simulink model "banc_test_bras_brushless_PF35_couronne_grande"  (R2025a)
settings: Solver=daessc  StartTime=0.0  StopTime=40  FixedStep=Ts  RelTol=1e-3  EnableMultiTasking=on
undefined symbols (not defined in the file or in its folder): Connection1, Connection10, Connection11, Connection12, Connection2, Connection3, Connection4, Connection5, Connection6, Connection7, Connection8, Connection9, X, Y, Z
libraries: sm_lib x16, nesl_utility x4
settings Model: Creator=vincp  LastModifiedBy=VincentPERRET
settings SolverCC: MaxConsecutiveMinStep=100  AllowMultiTaskInputOutput=on  ZeroCrossAlgorithm=Adaptive  PositivePriorityOrder=on
settings DataIOCC: ReturnWorkspaceOutputsName=tp821c331c_e25c_45d9_bd23_b4f1d96f521a
settings DebuggingCC: IgnoredZcDiagnostic=none
settings SFSimCC: SimTargetLang=C++  SimDLTargetLibrary=mkl-dnn
settings RTWCC: GPUComputeCapability=3.5
settings SimscapeCC: ExplicitSolverDiagnosticOptions=none  SimscapeLogName=simlog_ee_bldc_speed_control  SimscapeLogLimitData=off

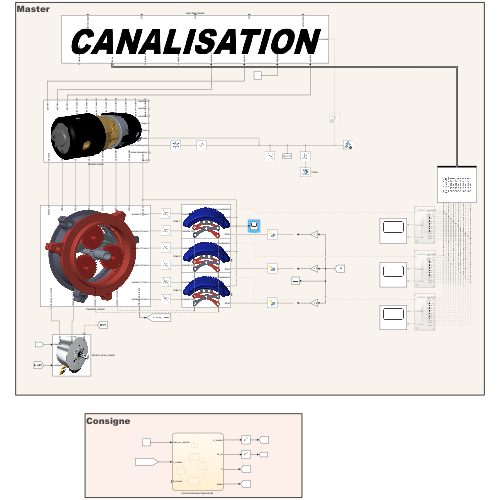
[thumbnail: Simulink's stored preview of the top-level diagram]
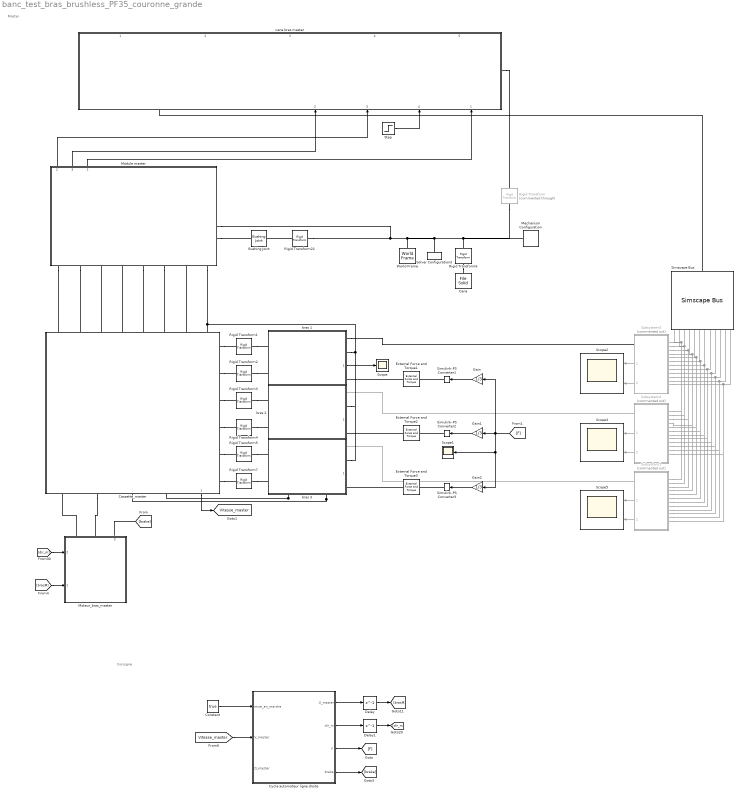
== system banc_test_bras_brushless_PF35_couronne_grande ==
  note: Consigne
  note: Master
  Bushing Joint : sm_lib/Joints/Bushing Joint  JointMode=Normal  CompositeWrenchDir=FollowerOnBase  CompositeWrenchFrame=BaseFrame  SenseConstraintForce=off  SenseConstraintTorque=off  SenseTotalForce=off  SenseTotalTorque=off  PxPositionTargetSpecify=off  PxPositionTargetPriority=High  PxPositionTargetValue=0  PxPositionTargetValueUnits=m  PxVelocityTargetSpecify=off  PxVelocityTargetPriority=High  PxVelocityTargetValue=0  PxVelocityTargetValueUnits=m/s  PxEquilibriumPosition=0  PxEquilibriumPositionUnits=m  PxSpringStiffness=0  PxSpringStiffnessUnits=N/m  PxDampingCoefficient=0  PxDampingCoefficientUnits=N/(m/s)  PxLowerLimitSpecify=off  PxLowerLimitBound=-1  PxLowerLimitBoundUnits=m  PxLowerLimitStiffness=1e6  PxLowerLimitStiffnessUnits=N/m  PxLowerLimitDamping=1e3  PxLowerLimitDampingUnits=N/(m/s)  PxLowerLimitTransitionRegionWidth=1e-4  PxLowerLimitTransitionRegionWidthUnits=m  PxUpperLimitSpecify=off  PxUpperLimitBound=1  PxUpperLimitBoundUnits=m  PxUpperLimitStiffness=1e6  PxUpperLimitStiffnessUnits=N/m  PxUpperLimitDamping=1e3  PxUpperLimitDampingUnits=N/(m/s)  PxUpperLimitTransitionRegionWidth=1e-4  PxUpperLimitTransitionRegionWidthUnits=m  PxTorqueActuationMode=NoTorque  PxMotionActuationMode=ComputedMotion  PxSensePosition=off  PxSenseVelocity=off  PxSenseAcceleration=off  PxSenseTorqueForce=off  PxSenseLowerLimitTorqueForce=off  PxSenseUpperLimitTorqueForce=off  PyPositionTargetSpecify=off  PyPositionTargetPriority=High  PyPositionTargetValue=0  PyPositionTargetValueUnits=m  PyVelocityTargetSpecify=off  PyVelocityTargetPriority=High  PyVelocityTargetValue=0  PyVelocityTargetValueUnits=m/s  PyEquilibriumPosition=0  PyEquilibriumPositionUnits=m  PySpringStiffness=0  PySpringStiffnessUnits=N/m  PyDampingCoefficient=0  PyDampingCoefficientUnits=N/(m/s)  PyLowerLimitSpecify=off  PyLowerLimitBound=-1  PyLowerLimitBoundUnits=m  PyLowerLimitStiffness=1e6  PyLowerLimitStiffnessUnits=N/m  PyLowerLimitDamping=1e3  PyLowerLimitDampingUnits=N/(m/s)  PyLowerLimitTransitionRegionWidth=1e-4  PyLowerLimitTransitionRegionWidthUnits=m  PyUpperLimitSpecify=off  PyUpperLimitBound=1  PyUpperLimitBoundUnits=m  PyUpperLimitStiffness=1e6  PyUpperLimitStiffnessUnits=N/m  PyUpperLimitDamping=1e3  PyUpperLimitDampingUnits=N/(m/s)  PyUpperLimitTransitionRegionWidth=1e-4  PyUpperLimitTransitionRegionWidthUnits=m  PyTorqueActuationMode=NoTorque  PyMotionActuationMode=ComputedMotion  PySensePosition=off  PySenseVelocity=off  PySenseAcceleration=off  PySenseTorqueForce=off  PySenseLowerLimitTorqueForce=off  PySenseUpperLimitTorqueForce=off  PzPositionTargetSpecify=off  PzPositionTargetPriority=High  PzPositionTargetValue=0  PzPositionTargetValueUnits=m  PzVelocityTargetSpecify=off  PzVelocityTargetPriority=High  PzVelocityTargetValue=-0.1  PzVelocityTargetValueUnits=m/s  PzEquilibriumPosition=0  PzEquilibriumPositionUnits=m  PzSpringStiffness=0  PzSpringStiffnessUnits=N/m  PzDampingCoefficient=0  PzDampingCoefficientUnits=N/(m/s)  PzLowerLimitSpecify=off  PzLowerLimitBound=-1  PzLowerLimitBoundUnits=m  PzLowerLimitStiffness=1e6  PzLowerLimitStiffnessUnits=N/m  PzLowerLimitDamping=1e3  PzLowerLimitDampingUnits=N/(m/s)  PzLowerLimitTransitionRegionWidth=1e-4  PzLowerLimitTransitionRegionWidthUnits=m  PzUpperLimitSpecify=off  PzUpperLimitBound=1  PzUpperLimitBoundUnits=m  PzUpperLimitStiffness=1e6  PzUpperLimitStiffnessUnits=N/m  PzUpperLimitDamping=1e3  PzUpperLimitDampingUnits=N/(m/s)  PzUpperLimitTransitionRegionWidth=1e-4  PzUpperLimitTransitionRegionWidthUnits=m  PzTorqueActuationMode=NoTorque  PzMotionActuationMode=ComputedMotion  PzSensePosition=off  PzSenseVelocity=off  PzSenseAcceleration=off  PzSenseTorqueForce=off  PzSenseLowerLimitTorqueForce=off  PzSenseUpperLimitTorqueForce=off  RxPositionTargetSpecify=off  RxPositionTargetPriority=High  RxPositionTargetValue=0  RxPositionTargetValueUnits=deg  RxVelocityTargetSpecify=off  RxVelocityTargetPriority=High  RxVelocityTargetValue=0  RxVelocityTargetValueUnits=deg/s  RxEquilibriumPosition=0  RxEquilibriumPositionUnits=deg  RxSpringStiffness=0  RxSpringStiffnessUnits=N*m/deg  RxDampingCoefficient=0  RxDampingCoefficientUnits=N*m/(deg/s)  RxLowerLimitSpecify=off  RxLowerLimitBound=-90  RxLowerLimitBoundUnits=deg  RxLowerLimitStiffness=1e4  RxLowerLimitStiffnessUnits=N*m/deg  RxLowerLimitDamping=10  RxLowerLimitDampingUnits=N*m/(deg/s)  RxLowerLimitTransitionRegionWidth=0.1  RxLowerLimitTransitionRegionWidthUnits=deg  RxUpperLimitSpecify=off  RxUpperLimitBound=90  RxUpperLimitBoundUnits=deg  RxUpperLimitStiffness=1e4  RxUpperLimitStiffnessUnits=N*m/deg  RxUpperLimitDamping=10  RxUpperLimitDampingUnits=N*m/(deg/s)  RxUpperLimitTransitionRegionWidth=0.1  RxUpperLimitTransitionRegionWidthUnits=deg  RxTorqueActuationMode=NoTorque  RxMotionActuationMode=ComputedMotion  RxSensePosition=off  RxSenseVelocity=off  RxSenseAcceleration=off  RxSenseTorqueForce=off  RxSenseLowerLimitTorqueForce=off  RxSenseUpperLimitTorqueForce=off  RyPositionTargetSpecify=off  RyPositionTargetPriority=High  RyPositionTargetValue=0  RyPositionTargetValueUnits=deg  RyVelocityTargetSpecify=off  RyVelocityTargetPriority=High  RyVelocityTargetValue=0  RyVelocityTargetValueUnits=deg/s  RyEquilibriumPosition=0  RyEquilibriumPositionUnits=deg  RySpringStiffness=0  RySpringStiffnessUnits=N*m/deg  RyDampingCoefficient=0  RyDampingCoefficientUnits=N*m/(deg/s)  RyLowerLimitSpecify=off  RyLowerLimitBound=-90  RyLowerLimitBoundUnits=deg  RyLowerLimitStiffness=1e4  RyLowerLimitStiffnessUnits=N*m/deg  RyLowerLimitDamping=10  RyLowerLimitDampingUnits=N*m/(deg/s)  RyLowerLimitTransitionRegionWidth=0.1  RyLowerLimitTransitionRegionWidthUnits=deg  RyUpperLimitSpecify=off  RyUpperLimitBound=90  RyUpperLimitBoundUnits=deg  RyUpperLimitStiffness=1e4  RyUpperLimitStiffnessUnits=N*m/deg  RyUpperLimitDamping=10  RyUpperLimitDampingUnits=N*m/(deg/s)  RyUpperLimitTransitionRegionWidth=0.1  RyUpperLimitTransitionRegionWidthUnits=deg  RyTorqueActuationMode=NoTorque  RyMotionActuationMode=ComputedMotion  RySensePosition=off  RySenseVelocity=off  RySenseAcceleration=off  RySenseTorqueForce=off  RySenseLowerLimitTorqueForce=off  RySenseUpperLimitTorqueForce=off  RzPositionTargetSpecify=off  RzPositionTargetPriority=High  RzPositionTargetValue=0  RzPositionTargetValueUnits=deg  RzVelocityTargetSpecify=off  RzVelocityTargetPriority=High  RzVelocityTargetValue=20  RzVelocityTargetValueUnits=deg/s  RzEquilibriumPosition=0  RzEquilibriumPositionUnits=deg  RzSpringStiffness=0  RzSpringStiffnessUnits=N*m/deg  RzDampingCoefficient=0  RzDampingCoefficientUnits=N*m/(deg/s)  RzLowerLimitSpecify=off  RzLowerLimitBound=-90  RzLowerLimitBoundUnits=deg  RzLowerLimitStiffness=1e4  RzLowerLimitStiffnessUnits=N*m/deg  RzLowerLimitDamping=10  RzLowerLimitDampingUnits=N*m/(deg/s)  RzLowerLimitTransitionRegionWidth=0.1  RzLowerLimitTransitionRegionWidthUnits=deg  RzUpperLimitSpecify=off  RzUpperLimitBound=90  RzUpperLimitBoundUnits=deg  RzUpperLimitStiffness=1e4  RzUpperLimitStiffnessUnits=N*m/deg  RzUpperLimitDamping=10  RzUpperLimitDampingUnits=N*m/(deg/s)  RzUpperLimitTransitionRegionWidth=0.1  RzUpperLimitTransitionRegionWidthUnits=deg  RzTorqueActuationMode=NoTorque  RzMotionActuationMode=ComputedMotion  RzSensePosition=off  RzSenseVelocity=off  RzSenseAcceleration=off  RzSenseTorqueForce=off  RzSenseLowerLimitTorqueForce=off  RzSenseUpperLimitTorqueForce=off
  Cana : sm_lib/Body Elements/File Solid  ExtGeomFileName=STEP\canalisation_350.obj  UnitType=Custom  ExtGeomFileUnits=m  StepReaderType=HEX  ExportConvexHullGeometry=off  InertiaType=CalculateFromGeometry  BasedOnType=Density  Density=0  DensityUnits=kg/m^3  Mass=1  MassUnits=kg  CenterOfMass=[0 0 0]  CenterOfMassUnits=m  MomentsOfInertia=[1 1 1]  MomentsOfInertiaUnits=kg*m^2  ProductsOfInertia=[0 0 0]  ProductsOfInertiaUnits=kg*m^2  GraphicType=FromGeometry  MarkerShape=Sphere  MarkerSize=10  GraphicVisPropType=SimpleVisualProperties  GraphicDiffuseColor=[0.8 0.8 0.8]  GraphicOpacity=0.4  GraphicSpecularColor=[0.5 0.5 0.5 1.0]  GraphicAmbientColor=[0.15 0.15 0.15 1.0]  GraphicEmissiveColor=[0.0 0.0 0.0 1.0]  GraphicShininess=75  DoExposeReferenceFrame=on  SerializedFrames=<Frames/>
  Cassette_master : Subsystem  ReferencedSubsystem=Cassette_bras_couronne_350
      settings: PortSchema="{\"entries\":[{\"content\":{\"sides\":[{\"content\":{\"connectorIds\":[\"LConn1\",\"LConn2\",\"LConn3\",\"LConn4\",\"LConn5\",\"LConn6\",\"LConn7\",\"LConn8\"]},\"type\":\"ConnectorPlacement.EquallySpacedRectSide\",\"uuid\":\"969d9e5a-e216-44d5-83f9-8c82118e2953\"},{\"content\":{\"connectorIds\":[\"RConn1\",\"RConn2\",\"RConn10\",\"RConn9\",\"Out1\"],\"side\":\"RIGHT\"},\"type\":\"ConnectorPlacement.EquallySpacedRectSide\",\"uuid\":\"1a9b204a-bf00-4ee8-bed5-7f81c593e67c\"},{\"content\":{\"side\":\"TOP\"},\"type\":\"ConnectorPlacement.EquallySpacedRectSide\",\"uuid\":\"a2c44173-d7f6-4154-9e72-3423cec1ec7c\"},{\"content\":{\"connectorIds\":[\"RConn3\",\"RConn4\",\"RConn5\",\"RConn6\",\"RConn7\",\"RConn8\"],\"side\":\"BOTTOM\"},\"type\":\"ConnectorPlacement.EquallySpacedRectSide\",\"uuid\":\"271c323f-6b2f-47cd-9b92-95e1b3728dfc\"}]},\"type\":\"ConnectorPlacement.EquallySpacedConnector\",\"uuid\":\"47e9a915-ac6c-453e-a781-819eb7e69896\"}],\"packageUris\":[\"http://schema.mathworks.com/mf0/Connector/R2020b\"],\"version\":\"1.0\"}"
  Constant : Constant  Value=true
  "Cycle automoteur ligne droite " : Stateflow chart  TreatAsAtomicUnit=on
  Delay : Delay  DelayLength=1
  Delay1 : Delay  DelayLength=1
  External Force and Torque1 : sm_lib/Forces and Torques/External Force and Torque  EnableForceX=off  EnableForceY=off  EnableForceZ=on  EnableForce=off  ForceResolutionFrame=World  EnableTorqueX=off  EnableTorqueY=off  EnableTorqueZ=off  EnableTorque=off  TorqueResolutionFrame=AttachedFrame
  External Force and Torque2 : sm_lib/Forces and Torques/External Force and Torque  EnableForceX=off  EnableForceY=off  EnableForceZ=on  EnableForce=off  ForceResolutionFrame=World  EnableTorqueX=off  EnableTorqueY=off  EnableTorqueZ=off  EnableTorque=off  TorqueResolutionFrame=AttachedFrame
  External Force and Torque3 : sm_lib/Forces and Torques/External Force and Torque  EnableForceX=off  EnableForceY=off  EnableForceZ=on  EnableForce=off  ForceResolutionFrame=World  EnableTorqueX=off  EnableTorqueY=off  EnableTorqueZ=off  EnableTorque=off  TorqueResolutionFrame=AttachedFrame
  Gain : Gain  Gain=1/3
  Gain1 : Gain  Gain=1/3
  Gain2 : Gain  Gain=1/3
  Mechanism Configuration : sm_lib/Utilities/Mechanism Configuration  UniformGravity=Constant  GravityVector=[0 0 0]  GravityVectorUnits=m/s^2  LinearizationDelta=0.001  JointModeTransitionNonlinearIterations=2
  Module master : Subsystem  ReferencedSubsystem=Module_master_
      settings: PortSchema="{\"entries\":[{\"content\":{\"sides\":[{\"content\":{},\"type\":\"ConnectorPlacement.EquallySpacedRectSide\",\"uuid\":\"3f3269b3-57e5-4234-824e-382e7f277697\"},{\"content\":{\"connectorIds\":[\"RConn1\",\"RConn2\",\"RConn3\",\"RConn4\",\"RConn23\",\"RConn13\",\"RConn5\",\"RConn24\",\"RConn25\"],\"side\":\"RIGHT\"},\"type\":\"ConnectorPlacement.EquallySpacedRectSide\",\"uuid\":\"0677a46d-6be2-4f10-aa29-3cc099f9cb16\"},{\"content\":{\"connectorIds\":[\"Out2\",\"Out3\",\"Out1\",\"RConn15\",\"RConn16\",\"RConn17\",\"RConn18\",\"RConn19\",\"RConn22\",\"RConn20\",\"RConn21\"],\"side\":\"TOP\"},\"type\":\"ConnectorPlacement.EquallySpacedRectSide\",\"uuid\":\"0416d965-f3e9-453f-90f5-e0573e577292\"},{\"content\":{\"connectorIds\":[\"RConn7\",\"RConn6\",\"RConn8\",\"RConn9\",\"RConn10\",\"RConn11\",\"RConn12\",\"RConn14\"],\"side\":\"BOTTOM\"},\"type\":\"ConnectorPlacement.EquallySpacedRectSide\",\"uuid\":\"ddd7c1c4-6c9f-4a33-95d1-c43d9c37bd43\"}]},\"type\":\"ConnectorPlacement.EquallySpacedConnector\",\"uuid\":\"6eeefed7-e4c2-43a4-8c68-979865c84a5f\"}],\"packageUris\":[\"http://schema.mathworks.com/mf0/Connector/R2020b\"],\"version\":\"1.0\"}"
  Moteur_bras_master : Subsystem  ReferencedSubsystem=moteur_bras
      settings: PortSchema="{\"entries\":[{\"content\":{\"sides\":[{\"content\":{},\"type\":\"ConnectorPlacement.EquallySpacedRectSide\",\"uuid\":\"44ca8511-91a9-4f9f-9d47-c484c720622d\"},{\"content\":{\"connectorIds\":[\"LConn1\",\"LConn2\",\"In3\"],\"side\":\"RIGHT\"},\"type\":\"ConnectorPlacement.EquallySpacedRectSide\",\"uuid\":\"a5d61267-f650-46c1-a6d3-db3818e00f2b\"},{\"content\":{\"connectorIds\":[\"In1\",\"In2\"],\"side\":\"TOP\"},\"type\":\"ConnectorPlacement.EquallySpacedRectSide\",\"uuid\":\"e67d56db-b7fc-4044-bce5-121564a75cb7\"},{\"content\":{\"side\":\"BOTTOM\"},\"type\":\"ConnectorPlacement.EquallySpacedRectSide\",\"uuid\":\"6d85dbd1-b9f4-47c6-b27b-ccd28f0623b4\"}]},\"type\":\"ConnectorPlacement.EquallySpacedConnector\",\"uuid\":\"493fcdaf-48cb-4fa3-bb99-5dc2bf522b32\"}],\"packageUris\":[\"http://schema.mathworks.com/mf0/Connector/R2020b\"],\"version\":\"1.0\"}"
  Rigid Transform : sm_lib/Frames and Transforms/Rigid Transform  Commented=through  RotationMethod=StandardAxis  FollAlignAxisA=+X  BaseAlignAxisA=+Y  FollAlignAxisB=+Y  BaseAlignAxisB=+Z  RotationStandardAxis=+X  RotationAngle=90  RotationAngleUnits=deg  RotationArbitraryAxis=[0 0 1]  RotationSequenceAxes=FollowerAxes  RotationSequence=XYX  RotationSequenceAngles=[0 0 0]  RotationSequenceAnglesUnits=deg  RotationMatrix=[1 0 0;0 1 0;0 0 1]  Quaternion=[1 0 0 0]  TranslationMethod=None  TranslationCartesianOffset=[0 0 0]  TranslationCartesianOffsetUnits=m  TranslationStandardAxis=+Z  TranslationStandardOffset=0  TranslationStandardOffsetUnits=m  TranslationROffset=0  TranslationROffsetUnits=m  TranslationThetaOffset=0  TranslationThetaOffsetUnits=deg  TranslationZOffset=0  TranslationZOffsetUnits=m
  Rigid Transform1 : sm_lib/Frames and Transforms/Rigid Transform  RotationMethod=StandardAxis  FollAlignAxisA=+X  BaseAlignAxisA=+Y  FollAlignAxisB=+Y  BaseAlignAxisB=+Z  RotationStandardAxis=-Z  RotationAngle=64  RotationAngleUnits=deg  RotationArbitraryAxis=[0 0 1]  RotationSequenceAxes=FollowerAxes  RotationSequence=XYX  RotationSequenceAngles=[0 0 0]  RotationSequenceAnglesUnits=deg  RotationMatrix=[1 0 0;0 1 0;0 0 1]  Quaternion=[1 0 0 0]  TranslationMethod=StandardAxis  TranslationCartesianOffset=[0 0 0]  TranslationCartesianOffsetUnits=m  TranslationStandardAxis=+Z  TranslationStandardOffset=5  TranslationStandardOffsetUnits=mm  TranslationROffset=0  TranslationROffsetUnits=m  TranslationThetaOffset=0  TranslationThetaOffsetUnits=deg  TranslationZOffset=0  TranslationZOffsetUnits=m
  Rigid Transform2 : sm_lib/Frames and Transforms/Rigid Transform  RotationMethod=StandardAxis  FollAlignAxisA=+X  BaseAlignAxisA=+Y  FollAlignAxisB=+Y  BaseAlignAxisB=+Z  RotationStandardAxis=+Z  RotationAngle=145  RotationAngleUnits=deg  RotationArbitraryAxis=[0 0 1]  RotationSequenceAxes=FollowerAxes  RotationSequence=XYX  RotationSequenceAngles=[0 0 0]  RotationSequenceAnglesUnits=deg  RotationMatrix=[1 0 0;0 1 0;0 0 1]  Quaternion=[1 0 0 0]  TranslationMethod=StandardAxis  TranslationCartesianOffset=[0 0 0]  TranslationCartesianOffsetUnits=m  TranslationStandardAxis=+Z  TranslationStandardOffset=5  TranslationStandardOffsetUnits=mm  TranslationROffset=0  TranslationROffsetUnits=m  TranslationThetaOffset=0  TranslationThetaOffsetUnits=deg  TranslationZOffset=0  TranslationZOffsetUnits=m
  Rigid Transform22 : sm_lib/Frames and Transforms/Rigid Transform  RotationMethod=RotationSequence  FollAlignAxisA=+X  BaseAlignAxisA=+Y  FollAlignAxisB=+Y  BaseAlignAxisB=+Z  RotationStandardAxis=+Z  RotationAngle=90  RotationAngleUnits=deg  RotationArbitraryAxis=[0 0 1]  RotationSequenceAxes=FollowerAxes  RotationSequence=ZYZ  RotationSequenceAngles=[90 180 0]  RotationSequenceAnglesUnits=deg  RotationMatrix=[1 0 0; 0 1 0; 0 0 1]  Quaternion=[1 0 0 0]  TranslationMethod=StandardAxis  TranslationCartesianOffset=[30 400 -450]  TranslationCartesianOffsetUnits=mm  TranslationStandardAxis=+Z  TranslationStandardOffset=500  TranslationStandardOffsetUnits=mm  TranslationROffset=0  TranslationROffsetUnits=m  TranslationThetaOffset=0  TranslationThetaOffsetUnits=deg  TranslationZOffset=0  TranslationZOffsetUnits=m
  Rigid Transform3 : sm_lib/Frames and Transforms/Rigid Transform  RotationMethod=StandardAxis  FollAlignAxisA=+X  BaseAlignAxisA=+Y  FollAlignAxisB=+Y  BaseAlignAxisB=+Z  RotationStandardAxis=+Z  RotationAngle=150  RotationAngleUnits=deg  RotationArbitraryAxis=[0 0 1]  RotationSequenceAxes=FollowerAxes  RotationSequence=XYX  RotationSequenceAngles=[0 0 0]  RotationSequenceAnglesUnits=deg  RotationMatrix=[1 0 0;0 1 0;0 0 1]  Quaternion=[1 0 0 0]  TranslationMethod=StandardAxis  TranslationCartesianOffset=[0 0 0]  TranslationCartesianOffsetUnits=m  TranslationStandardAxis=+Z  TranslationStandardOffset=5  TranslationStandardOffsetUnits=mm  TranslationROffset=0  TranslationROffsetUnits=m  TranslationThetaOffset=0  TranslationThetaOffsetUnits=deg  TranslationZOffset=0  TranslationZOffsetUnits=m
  Rigid Transform4 : sm_lib/Frames and Transforms/Rigid Transform  RotationMethod=StandardAxis  FollAlignAxisA=+X  BaseAlignAxisA=+Y  FollAlignAxisB=+Y  BaseAlignAxisB=+Z  RotationStandardAxis=-Z  RotationAngle=60  RotationAngleUnits=deg  RotationArbitraryAxis=[0 0 1]  RotationSequenceAxes=FollowerAxes  RotationSequence=XYX  RotationSequenceAngles=[0 0 0]  RotationSequenceAnglesUnits=deg  RotationMatrix=[1 0 0;0 1 0;0 0 1]  Quaternion=[1 0 0 0]  TranslationMethod=StandardAxis  TranslationCartesianOffset=[0 0 0]  TranslationCartesianOffsetUnits=m  TranslationStandardAxis=+Z  TranslationStandardOffset=5  TranslationStandardOffsetUnits=mm  TranslationROffset=0  TranslationROffsetUnits=m  TranslationThetaOffset=0  TranslationThetaOffsetUnits=deg  TranslationZOffset=0  TranslationZOffsetUnits=m
  Rigid Transform5 : sm_lib/Frames and Transforms/Rigid Transform  RotationMethod=StandardAxis  FollAlignAxisA=+X  BaseAlignAxisA=+Y  FollAlignAxisB=+Y  BaseAlignAxisB=+Z  RotationStandardAxis=-Z  RotationAngle=90  RotationAngleUnits=deg  RotationArbitraryAxis=[0 0 1]  RotationSequenceAxes=FollowerAxes  RotationSequence=XYX  RotationSequenceAngles=[0 0 0]  RotationSequenceAnglesUnits=deg  RotationMatrix=[1 0 0;0 1 0;0 0 1]  Quaternion=[1 0 0 0]  TranslationMethod=StandardAxis  TranslationCartesianOffset=[0 0 0]  TranslationCartesianOffsetUnits=m  TranslationStandardAxis=+Z  TranslationStandardOffset=5  TranslationStandardOffsetUnits=mm  TranslationROffset=0  TranslationROffsetUnits=m  TranslationThetaOffset=0  TranslationThetaOffsetUnits=deg  TranslationZOffset=0  TranslationZOffsetUnits=m
  Rigid Transform6 : sm_lib/Frames and Transforms/Rigid Transform  RotationMethod=None  FollAlignAxisA=+X  BaseAlignAxisA=+Y  FollAlignAxisB=+Y  BaseAlignAxisB=+Z  RotationStandardAxis=+Y  RotationAngle=180  RotationAngleUnits=deg  RotationArbitraryAxis=[0 0 1]  RotationSequenceAxes=FollowerAxes  RotationSequence=XYX  RotationSequenceAngles=[0 0 0]  RotationSequenceAnglesUnits=deg  RotationMatrix=[1 0 0;0 1 0;0 0 1]  Quaternion=[1 0 0 0]  TranslationMethod=None  TranslationCartesianOffset=[-400 0 -500]  TranslationCartesianOffsetUnits=mm  TranslationStandardAxis=+Z  TranslationStandardOffset=0  TranslationStandardOffsetUnits=m  TranslationROffset=0  TranslationROffsetUnits=m  TranslationThetaOffset=0  TranslationThetaOffsetUnits=deg  TranslationZOffset=0  TranslationZOffsetUnits=m
  Rigid Transform7 : sm_lib/Frames and Transforms/Rigid Transform  RotationMethod=StandardAxis  FollAlignAxisA=+X  BaseAlignAxisA=+Y  FollAlignAxisB=+Y  BaseAlignAxisB=+Z  RotationStandardAxis=+Z  RotationAngle=180  RotationAngleUnits=deg  RotationArbitraryAxis=[0 0 1]  RotationSequenceAxes=FollowerAxes  RotationSequence=XYX  RotationSequenceAngles=[0 0 0]  RotationSequenceAnglesUnits=deg  RotationMatrix=[1 0 0;0 1 0;0 0 1]  Quaternion=[1 0 0 0]  TranslationMethod=StandardAxis  TranslationCartesianOffset=[0 0 0]  TranslationCartesianOffsetUnits=m  TranslationStandardAxis=+Z  TranslationStandardOffset=5  TranslationStandardOffsetUnits=mm  TranslationROffset=0  TranslationROffsetUnits=m  TranslationThetaOffset=0  TranslationThetaOffsetUnits=deg  TranslationZOffset=0  TranslationZOffsetUnits=m
  Scope : Scope
      settings: ActiveDisplayYMinimum=0.19535051101049178  ActiveDisplayYMaximum=0.19709732540962827  DataLoggingVariableName=ScopeData4
  Scope1 : Scope
      settings: ActiveDisplayYMinimum=-0.625  ActiveDisplayYMaximum=5.625  DataLoggingVariableName=ScopeData48
  Scope2 : Scope  NumInputPorts=2
      settings: ActiveDisplayYMinimum=37.43299350945631  ActiveDisplayYMaximum=101.90092677574211  DataLoggingVariableName=ScopeData49
  Scope3 : Scope  NumInputPorts=2
      settings: ActiveDisplayYMinimum=-32.07489  ActiveDisplayYMaximum=288.67405  DataLoggingVariableName=ScopeData50
  Scope5 : Scope  NumInputPorts=2
      settings: ActiveDisplayYMinimum=-32.07489  ActiveDisplayYMaximum=288.67405  DataLoggingVariableName=ScopeData31
  Simscape Bus : SimscapeBus  HierarchyStrings=Connection12;Connection11;Connection10;Connection9;Connection8;Connection7;Connection6;Connection5;Connection4;Connection3;Connection2;Connection1
  Simulink-PS Converter1 : nesl_utility/Simulink-PS Converter  PhysicalDomain=network_engine_domain  SubClassName=ps_input  LeftPortType=input  RightPortType=output  PseudoPeriodic=off  Frequencies=[]  NoiseDistribution=none  NoiseParameters=[]  Unit=1  AffineConversion=off  FilteringAndDerivatives=provide  SimscapeFilterOrder=1  InputFilterTimeConstant=0.001  UdotUserProvided=0
  Simulink-PS Converter2 : nesl_utility/Simulink-PS Converter  PhysicalDomain=network_engine_domain  SubClassName=ps_input  LeftPortType=input  RightPortType=output  PseudoPeriodic=off  Frequencies=[]  NoiseDistribution=none  NoiseParameters=[]  Unit=1  AffineConversion=off  FilteringAndDerivatives=provide  SimscapeFilterOrder=1  InputFilterTimeConstant=0.001  UdotUserProvided=0
  Simulink-PS Converter3 : nesl_utility/Simulink-PS Converter  PhysicalDomain=network_engine_domain  SubClassName=ps_input  LeftPortType=input  RightPortType=output  PseudoPeriodic=off  Frequencies=[]  NoiseDistribution=none  NoiseParameters=[]  Unit=1  AffineConversion=off  FilteringAndDerivatives=provide  SimscapeFilterOrder=1  InputFilterTimeConstant=0.001  UdotUserProvided=0
  Solver Configuration3 : nesl_utility/Solver Configuration  PhysicalDomain=network_engine_domain  SubClassName=solver  LeftPortType=input  RightPortType=generic  Tones=[]  Harmonics=[]  SimulateNoise=off  Profile=off  UseLocalSampling=off  EnableSwitchedLinearOptims=on  FrequencyDomain=off  UseCCode=off  RelTol=0.001  AbsTol=1e-06  MinStep=1e-09  ToWorkspace=off  RevertToSquareIcSolve=off  NumHomotopyIterations=100  PhasorMode=off  PhasorModeNumHarmonics=1  ConsistencySolver=NEWTON_FTOL  IndexReductionMethod=DerivativeReplacement  DoDC=off  ResidualTolerance=1e-3  ConsistencyTolSource=GLOBAL  ConsistencyAbsTol=0.001  ConsistencyRelTol=0.001  ConsistencyTolFactor=0.001  UseLocalSolver=off  LocalSolverChoice=NE_TRAPEZOIDAL_ADVANCER  ResolveIndetEquations=on  FunctionEvalNumThread=1  LocalSolverSampleTime=Ts  DoFixedCost=off  MaxNonlinIter=4  MaxModeIter=2  ComputeImpulses=off  ImpulseIterations=2  LinearAlgebra=auto  LinearAlgebraNumThread=0  EquationFormulation=NE_TIME_EF  DelaysMemoryBudget=1024  AutomaticFiltering=on  FilteringTimeConstant=0.01  PartitionStorageMethod=AS_NEEDED  PartitionMemoryBudget=1024  PartitionMethod=FAST  MultibodyUseLocalSolver=off  MultibodyLocalSolverChoice=ODE2  MultibodyLocalSolverSampleTime=0.0001
  Step : Step  Before=1  After=-1  SampleTime=0
  Subsystem3 : Subsystem  Commented=on  ReferencedSubsystem=contact_canalisation
      settings: PortSchema="{\"entries\":[{\"content\":{\"sides\":[{\"content\":{\"connectorIds\":[\"LConn12\",\"LConn11\",\"LConn10\",\"LConn7\",\"LConn9\",\"LConn8\",\"LConn4\",\"LConn3\",\"LConn1\",\"LConn5\",\"LConn2\",\"LConn6\"]},\"type\":\"ConnectorPlacement.EquallySpacedRectSide\",\"uuid\":\"cc6127df-d397-4b4c-ac82-4f83742e775e\"},{\"content\":{\"connectorIds\":[\"RConn1\",\"Out1\",\"Out2\"],\"side\":\"RIGHT\"},\"type\":\"ConnectorPlacement.EquallySpacedRectSide\",\"uuid\":\"98ad7edc-f29b-4da9-929d-5bdc04e492d8\"},{\"content\":{\"side\":\"TOP\"},\"type\":\"ConnectorPlacement.EquallySpacedRectSide\",\"uuid\":\"48ed23b2-0d62-4270-aaff-d987eb6b21c1\"}]},\"type\":\"ConnectorPlacement.EquallySpacedConnector\",\"uuid\":\"4be7faf1-9e2f-424b-9dfe-c6fda2353607\"}],\"packageUris\":[\"http://schema.mathworks.com/mf0/Connector/R2020b\"],\"version\":\"1.0\"}"
  Subsystem4 : Subsystem  Commented=on  ReferencedSubsystem=contact_canalisation
      settings: PortSchema="{\"entries\":[{\"content\":{\"sides\":[{\"content\":{\"connectorIds\":[\"LConn12\",\"LConn11\",\"LConn10\",\"LConn7\",\"LConn9\",\"LConn8\",\"LConn4\",\"LConn3\",\"LConn1\",\"LConn5\",\"LConn2\",\"LConn6\"]},\"type\":\"ConnectorPlacement.EquallySpacedRectSide\",\"uuid\":\"cc6127df-d397-4b4c-ac82-4f83742e775e\"},{\"content\":{\"connectorIds\":[\"RConn1\",\"Out1\",\"Out2\"],\"side\":\"RIGHT\"},\"type\":\"ConnectorPlacement.EquallySpacedRectSide\",\"uuid\":\"98ad7edc-f29b-4da9-929d-5bdc04e492d8\"},{\"content\":{\"side\":\"TOP\"},\"type\":\"ConnectorPlacement.EquallySpacedRectSide\",\"uuid\":\"48ed23b2-0d62-4270-aaff-d987eb6b21c1\"}]},\"type\":\"ConnectorPlacement.EquallySpacedConnector\",\"uuid\":\"4be7faf1-9e2f-424b-9dfe-c6fda2353607\"}],\"packageUris\":[\"http://schema.mathworks.com/mf0/Connector/R2020b\"],\"version\":\"1.0\"}"
  Subsystem5 : Subsystem  Commented=on  ReferencedSubsystem=contact_canalisation
      settings: PortSchema="{\"entries\":[{\"content\":{\"sides\":[{\"content\":{\"connectorIds\":[\"LConn12\",\"LConn11\",\"LConn10\",\"LConn7\",\"LConn9\",\"LConn8\",\"LConn4\",\"LConn3\",\"LConn1\",\"LConn5\",\"LConn2\",\"LConn6\"]},\"type\":\"ConnectorPlacement.EquallySpacedRectSide\",\"uuid\":\"cc6127df-d397-4b4c-ac82-4f83742e775e\"},{\"content\":{\"connectorIds\":[\"RConn1\",\"Out1\",\"Out2\"],\"side\":\"RIGHT\"},\"type\":\"ConnectorPlacement.EquallySpacedRectSide\",\"uuid\":\"98ad7edc-f29b-4da9-929d-5bdc04e492d8\"},{\"content\":{\"side\":\"TOP\"},\"type\":\"ConnectorPlacement.EquallySpacedRectSide\",\"uuid\":\"48ed23b2-0d62-4270-aaff-d987eb6b21c1\"}]},\"type\":\"ConnectorPlacement.EquallySpacedConnector\",\"uuid\":\"4be7faf1-9e2f-424b-9dfe-c6fda2353607\"}],\"packageUris\":[\"http://schema.mathworks.com/mf0/Connector/R2020b\"],\"version\":\"1.0\"}"
  World Frame : sm_lib/Frames and Transforms/World Frame
  bras 1 : Subsystem  ReferencedSubsystem=bras_PF25
      settings: PortSchema="{\"entries\":[{\"content\":{\"sides\":[{\"content\":{\"connectorIds\":[\"LConn1\",\"LConn2\"]},\"type\":\"ConnectorPlacement.EquallySpacedRectSide\",\"uuid\":\"53626720-9958-4ac4-88fa-52286cdb44da\"},{\"content\":{\"connectorIds\":[\"RConn1\",\"RConn3\",\"Out1\",\"RConn2\"],\"side\":\"RIGHT\"},\"type\":\"ConnectorPlacement.EquallySpacedRectSide\",\"uuid\":\"d018ad60-66d5-4743-b42a-577809bc0579\"},{\"content\":{\"side\":\"TOP\"},\"type\":\"ConnectorPlacement.EquallySpacedRectSide\",\"uuid\":\"f6880afb-2347-41d1-80ca-35463b8d5594\"},{\"content\":{\"connectorIds\":[\"LConn3\",\"LConn4\"],\"side\":\"BOTTOM\"},\"type\":\"ConnectorPlacement.EquallySpacedRectSide\",\"uuid\":\"2208f488-e347-4a6f-b702-dbdd4177085b\"}]},\"type\":\"ConnectorPlacement.EquallySpacedConnector\",\"uuid\":\"14ba9021-6286-4223-99de-985beb2c3192\"}],\"packageUris\":[\"http://schema.mathworks.com/mf0/Connector/R2020b\"],\"version\":\"1.0\"}"
  bras 2 : Subsystem  ReferencedSubsystem=bras_PF25
      settings: PortSchema="{\"entries\":[{\"content\":{\"sides\":[{\"content\":{\"connectorIds\":[\"LConn1\",\"LConn2\"]},\"type\":\"ConnectorPlacement.EquallySpacedRectSide\",\"uuid\":\"53626720-9958-4ac4-88fa-52286cdb44da\"},{\"content\":{\"connectorIds\":[\"RConn1\",\"RConn3\",\"Out1\",\"RConn2\"],\"side\":\"RIGHT\"},\"type\":\"ConnectorPlacement.EquallySpacedRectSide\",\"uuid\":\"d018ad60-66d5-4743-b42a-577809bc0579\"},{\"content\":{\"side\":\"TOP\"},\"type\":\"ConnectorPlacement.EquallySpacedRectSide\",\"uuid\":\"f6880afb-2347-41d1-80ca-35463b8d5594\"},{\"content\":{\"connectorIds\":[\"LConn3\",\"LConn4\"],\"side\":\"BOTTOM\"},\"type\":\"ConnectorPlacement.EquallySpacedRectSide\",\"uuid\":\"3279e7a6-d094-44d5-9c67-dd5fe60e7fc4\"}]},\"type\":\"ConnectorPlacement.EquallySpacedConnector\",\"uuid\":\"14ba9021-6286-4223-99de-985beb2c3192\"}],\"packageUris\":[\"http://schema.mathworks.com/mf0/Connector/R2020b\"],\"version\":\"1.0\"}"
  bras 3 : Subsystem  ReferencedSubsystem=bras_PF25
      settings: PortSchema="{\"entries\":[{\"content\":{\"sides\":[{\"content\":{\"connectorIds\":[\"LConn1\",\"LConn2\"]},\"type\":\"ConnectorPlacement.EquallySpacedRectSide\",\"uuid\":\"53626720-9958-4ac4-88fa-52286cdb44da\"},{\"content\":{\"connectorIds\":[\"RConn1\",\"RConn3\",\"Out1\",\"RConn2\"],\"side\":\"RIGHT\"},\"type\":\"ConnectorPlacement.EquallySpacedRectSide\",\"uuid\":\"d018ad60-66d5-4743-b42a-577809bc0579\"},{\"content\":{\"side\":\"TOP\"},\"type\":\"ConnectorPlacement.EquallySpacedRectSide\",\"uuid\":\"f6880afb-2347-41d1-80ca-35463b8d5594\"},{\"content\":{\"connectorIds\":[\"LConn3\",\"LConn4\"],\"side\":\"BOTTOM\"},\"type\":\"ConnectorPlacement.EquallySpacedRectSide\",\"uuid\":\"e33bcce5-ca5f-4dfb-b9c4-c76ffdb8cf78\"}]},\"type\":\"ConnectorPlacement.EquallySpacedConnector\",\"uuid\":\"14ba9021-6286-4223-99de-985beb2c3192\"}],\"packageUris\":[\"http://schema.mathworks.com/mf0/Connector/R2020b\"],\"version\":\"1.0\"}"
  cana bras master : Subsystem  LoadFcn=Parametre.m  ReferencedSubsystem=canalisation_suiveuse
      settings: PortSchema="{\"entries\":[{\"content\":{\"sides\":[{\"content\":{\"connectorIds\":[\"LConn1\",\"LConn2\",\"LConn3\",\"LConn4\",\"In2\",\"In3\",\"In4\",\"In1\"]},\"type\":\"ConnectorPlacement.EquallySpacedRectSide\",\"uuid\":\"57cdd168-7b90-44c2-9827-aab20de5ce30\"},{\"content\":{\"connectorIds\":[\"Out1\",\"Out2\",\"Out3\",\"Out4\",\"Out5\"],\"side\":\"RIGHT\"},\"type\":\"ConnectorPlacement.EquallySpacedRectSide\",\"uuid\":\"f21311ea-e7f6-4a31-b20e-9f1de8a9dc33\"},{\"content\":{\"side\":\"TOP\"},\"type\":\"ConnectorPlacement.EquallySpacedRectSide\",\"uuid\":\"f5efbfa1-6656-42d8-b800-0b73b1dfceb6\"},{\"content\":{\"connectorIds\":[\"RConn1\"],\"side\":\"BOTTOM\"},\"type\":\"ConnectorPlacement.EquallySpacedRectSide\",\"uuid\":\"c9b6144a-7869-4a60-96ee-1f643c516341\"}]},\"type\":\"ConnectorPlacement.EquallySpacedConnector\",\"uuid\":\"3e5878c9-89bc-4e86-b797-468e274615bc\"}],\"packageUris\":[\"http://schema.mathworks.com/mf0/Connector/R2020b\"],\"version\":\"1.0\"}"
  tag scope: Vitesse_master=global
  wires:
  "Cycle automoteur ligne droite "/4(brake) -> [brake]
  "Cycle automoteur ligne droite "/3(F) -> [F]
  [Vitesse_master] -> "Cycle automoteur ligne droite "/2(V_master)
  Delay1/1 -> [dir_m]
  Delay/1 -> [brasM]
  Module master/2 -> cana bras master/3
  Step/1 -> cana bras master/4
  Module master/1 -> cana bras master/1
  Module master/3 -> cana bras master/2
  [dir_m] -> Moteur_bras_master/2
  "Cycle automoteur ligne droite "/2(dir_m) -> Delay1/1
  Cassette_master/1 -> [Vitesse_master]
  [brasM] -> Moteur_bras_master/1
  Constant/1 -> "Cycle automoteur ligne droite "/1(mise_en_marche)
  "Cycle automoteur ligne droite "/1(U_master) -> Delay/1
  [F] -> Gain1/1, Gain2/1, Scope1/1, Gain/1
  Gain/1 -> Simulink-PS Converter1/1
  Gain2/1 -> Simulink-PS Converter3/1
  Gain1/1 -> Simulink-PS Converter2/1
  Subsystem3/1 -> Scope2/1
  Subsystem3/2 -> Scope2/2
  Subsystem4/1 -> Scope3/1
  Subsystem4/2 -> Scope3/2
  Subsystem5/1 -> Scope5/1
  Subsystem5/2 -> Scope5/2
  [brake] -> ?
  bras 1/1 -> Scope/1
  connections:
  Subsystem3/LConn6 -- Subsystem5/LConn6 -- Subsystem4/LConn6 -- Simscape Bus/LConn12
  Subsystem3/LConn2 -- Subsystem5/LConn2 -- Subsystem4/LConn2 -- Simscape Bus/LConn11
  Subsystem3/LConn5 -- Subsystem5/LConn5 -- Subsystem4/LConn5 -- Simscape Bus/LConn10
  Subsystem3/LConn1 -- Subsystem5/LConn1 -- Subsystem4/LConn1 -- Simscape Bus/LConn9
  Subsystem3/LConn3 -- Subsystem5/LConn3 -- Subsystem4/LConn3 -- Simscape Bus/LConn8
  Subsystem3/LConn4 -- Subsystem5/LConn4 -- Subsystem4/LConn4 -- Simscape Bus/LConn7
  Subsystem3/LConn8 -- Subsystem5/LConn8 -- Subsystem4/LConn8 -- Simscape Bus/LConn6
  Subsystem3/LConn9 -- Subsystem5/LConn9 -- Subsystem4/LConn9 -- Simscape Bus/LConn5
  Subsystem3/LConn7 -- Subsystem5/LConn7 -- Subsystem4/LConn7 -- Simscape Bus/LConn4
  Subsystem3/LConn10 -- Subsystem5/LConn10 -- Subsystem4/LConn10 -- Simscape Bus/LConn3
  Subsystem3/LConn11 -- Subsystem5/LConn11 -- Subsystem4/LConn11 -- Simscape Bus/LConn2
  Subsystem3/LConn12 -- Subsystem5/LConn12 -- Subsystem4/LConn12 -- Simscape Bus/LConn1
  Module master/RConn6 -- Cassette_master/LConn2
  Cassette_master/LConn3 -- Module master/RConn8
  Cassette_master/LConn4 -- Module master/RConn9
  Module master/RConn10 -- Cassette_master/LConn5
  Module master/RConn11 -- Cassette_master/LConn6
  Cassette_master/LConn7 -- Module master/RConn12
  Cassette_master/RConn8 -- Rigid Transform7/RConn1
  Cassette_master/RConn7 -- Rigid Transform5/RConn1
  Cassette_master/RConn6 -- Rigid Transform4/RConn1
  Cassette_master/RConn5 -- Rigid Transform3/RConn1
  Rigid Transform2/LConn1 -- bras 1/LConn2
  Rigid Transform1/LConn1 -- bras 1/LConn1
  Cassette_master/RConn2 -- Moteur_bras_master/LConn2
  Simscape Bus/RConn1 -- cana bras master/LConn2
  Moteur_bras_master/LConn1 -- Cassette_master/RConn1
  cana bras master/RConn1 -- Rigid Transform/RConn1
  Subsystem4/RConn1 -- bras 2/RConn1
  bras 1/RConn1 -- Subsystem3/RConn1
  Subsystem5/RConn1 -- bras 3/RConn1
  Rigid Transform7/LConn1 -- bras 3/LConn2
  Rigid Transform5/LConn1 -- bras 3/LConn1
  Rigid Transform4/LConn1 -- bras 2/LConn2
  Rigid Transform3/LConn1 -- bras 2/LConn1
  Cassette_master/RConn4 -- Rigid Transform2/RConn1
  Cassette_master/RConn3 -- Rigid Transform1/RConn1
  Rigid Transform22/RConn1 -- Bushing Joint/LConn1
  Rigid Transform6/RConn1 -- Cana/RConn1
  Module master/RConn5 -- Bushing Joint/RConn1
  Module master/RConn14 -- bras 3/RConn3 -- bras 2/RConn3 -- bras 1/RConn3 -- Cassette_master/LConn8
  Module master/RConn7 -- Cassette_master/LConn1
  Module master/RConn13 -- Rigid Transform/LConn1 -- Mechanism Configuration/RConn1 -- Rigid Transform6/LConn1 -- Solver Configuration3/RConn1 -- World Frame/RConn1 -- Rigid Transform22/LConn1
  Simulink-PS Converter2/RConn1 -- External Force and Torque2/LConn1
  External Force and Torque2/RConn1 -- bras 2/RConn2
  Simulink-PS Converter3/RConn1 -- External Force and Torque3/LConn1
  Simulink-PS Converter1/RConn1 -- External Force and Torque1/LConn1
  External Force and Torque3/RConn1 -- bras 3/RConn2
  External Force and Torque1/RConn1 -- bras 1/RConn2
  bras 3/LConn3 -- bras 1/LConn3 -- bras 2/LConn3 -- Cassette_master/RConn9
  bras 3/LConn4 -- bras 1/LConn4 -- bras 2/LConn4 -- Cassette_master/RConn10

== stateflow chart banc_test_bras_brushless_PF35_couronne_grande/Cycle automoteur ligne droite  ==
  state Attente
  state Deploiment_Master
    entry :
    U_master = 1200;
    dir_m = 0 ;
    brake=0
  state delay
    entry :
    U_master=1200;
    F=0;
  state delay1
    entry :
    U_master=1200;
    brake=0;
  state Retrait_Master
    entry :
    U_master = 1200;
    dir_m = 10 ;
    F=0;
  (default) -> Attente : {U_master=0 ;  dir_m=0;F=0 }
  Attente -> Deploiment_Master : [mise_en_marche & after(1,sec)]
  Deploiment_Master -> delay : [after(2,sec) & abs(V_master)<=0.005]
  delay1 -> Deploiment_Master : [after(1.5,sec)]
  delay -> Retrait_Master : [after(1.5,sec)]
  Retrait_Master -> delay1 : [after(2,sec) & abs(V_master)<=0.005]
  data: U_master output; mise_en_marche input; V_master input; D_master input; dir_m output; F output; brake output
